simulink model "eulerAnglePropagate"  (R2023b)
settings: Solver=VariableStepAuto  StartTime=0.0  StopTime=Tfinal  RelTol=1e-3
model workspace (MAT data in the model file):
  sequence = "313"
  u0 = [2.91319105247; 0.437912021527; 0.275895246399]
settings Model: Creator=stanforduser  LastModifiedBy=kristopherriordan
settings DataIOCC: ReturnWorkspaceOutputs=off

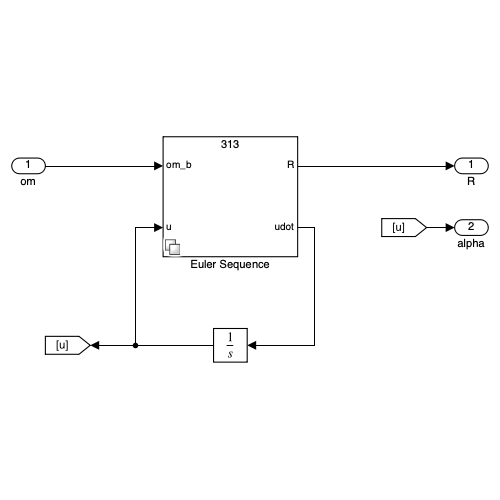
[thumbnail: Simulink's stored preview of the top-level diagram]
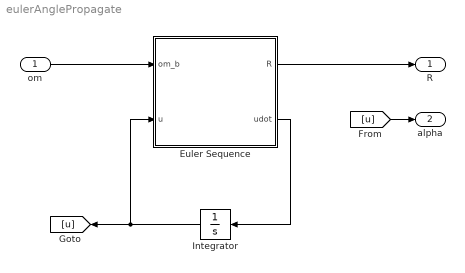
== system eulerAnglePropagate ==
  om : Inport
  Euler Sequence : Subsystem  Variant=on  VariantControl=313
  Integrator : Integrator  InitialCondition=u0
  R : Outport
  alpha : Outport  Port=2
  wires:
  Integrator/1 -> [u], Euler Sequence/2(u)
  om/1 -> Euler Sequence/1(om_b)
  Euler Sequence/1(R) -> R/1
  Euler Sequence/2(udot) -> Integrator/1
  [u] -> alpha/1

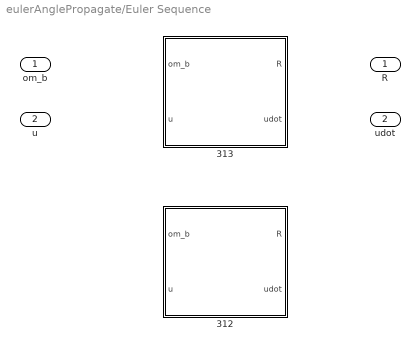
== system eulerAnglePropagate/Euler Sequence ==
  om_b : Inport
  u : Inport  Port=2
  312 : Subsystem  VariantControl="sequence==\"312\""
  313 : Subsystem  VariantControl="sequence==\"313\""
  R : Outport
  udot : Outport  Port=2

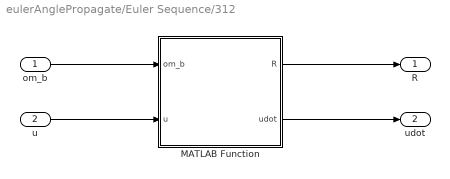
== system eulerAnglePropagate/Euler Sequence/312 ==
  om_b : Inport
  u : Inport  Port=2
  MATLAB Function : MATLAB Function  TreatAsAtomicUnit=on
  R : Outport
  udot : Outport  Port=2
  wires:
  MATLAB Function/1(R) -> R/1
  u/1 -> MATLAB Function/2(u)
  MATLAB Function/2(udot) -> udot/1
  om_b/1 -> MATLAB Function/1(om_b)

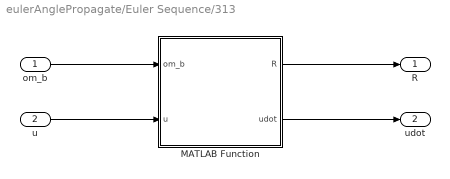
== system eulerAnglePropagate/Euler Sequence/313 ==
  om_b : Inport
  u : Inport  Port=2
  MATLAB Function : MATLAB Function  TreatAsAtomicUnit=on
  R : Outport
  udot : Outport  Port=2
  wires:
  MATLAB Function/1(R) -> R/1
  u/1 -> MATLAB Function/2(u)
  MATLAB Function/2(udot) -> udot/1
  om_b/1 -> MATLAB Function/1(om_b)

== matlab function eulerAnglePropagate/Euler Sequence/313/MATLAB Function ==
  data: om_b input size=[3 1]; u input size=[3 1]; R output; udot output size=[3 1]
function [R, udot] = eulerAnglePropagate(om_b, u)

% udot = zeros(size(u));

phi = u(1);
theta = u(2);
psi = u(3);

E_prime_inv = (1/sin(theta)) .* [-sin(phi)*cos(theta), -cos(phi)*cos(theta), sin(theta);
                                cos(phi)*sin(theta), -sin(phi)*sin(theta), 0;
                                sin(phi), cos(phi), 0];

udot = E_prime_inv*om_b;


R = [cos(phi)*cos(psi) - sin(phi)*cos(theta)*sin(psi) , cos(phi)*sin(psi) + sin(phi)*cos(theta)*cos(psi), sin(phi)*sin(theta);
    -sin(phi)*cos(psi) - cos(phi)*cos(theta)*sin(psi), -sin(phi)*sin(psi) + cos(phi)*cos(theta)*cos(psi), cos(phi)*sin(theta);
    sin(theta)*sin(psi), -sin(theta)*cos(psi), cos(theta)];

== matlab function eulerAnglePropagate/Euler Sequence/312/MATLAB Function ==
  data: om_b input size=[3 1]; u input size=[3 1]; R output; udot output size=[3 1]
function [R, udot] = eulerAnglePropagate(om_b, u)

% udot = zeros(size(u));

phi = u(1);
theta = u(2);
psi = u(3);

E_prime_inv = (1/cos(theta)) .* [sin(phi)*sin(theta), cos(phi)*sin(theta), cos(theta);
                                cos(theta)*cos(phi), -sin(phi)*cos(theta), 0;
                                sin(phi), cos(phi), 0];

udot = E_prime_inv*om_b;


R = [cos(phi)*cos(psi) + sin(phi)*sin(theta)*sin(psi), sin(phi)*cos(theta), -cos(phi)*sin(psi) + sin(phi)*sin(theta)*cos(psi);
    -sin(phi)*cos(psi) + cos(phi)*sin(theta)*sin(psi), cos(theta)*cos(phi), sin(phi)*sin(psi) + cos(phi)*sin(theta)*cos(psi);
    cos(theta)*sin(psi), -sin(theta), cos(theta)*cos(psi)];
